simulink model "Transform"  (R2017a)
settings: Solver=VariableStepAuto  StartTime=0.0  StopTime=10.0  MaxStep=0.01  RelTol=1e-3
settings Model: Creator=drone  LastModifiedBy=drone

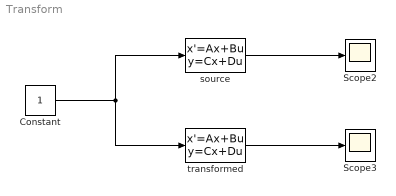
== system Transform ==
  Constant : Constant
  Scope2 : Scope
  Scope3 : Scope
  source : StateSpace  A=[0.5 -10; 1 -2]  B=[0; 1]  C=[3 1]  D=0  X0=0
  transformed : StateSpace  A=[5.5 -1.25; 38 -7]  B=[0; 2]  C=[10 0.5]  D=0  X0=0
  wires:
  Constant/1 -> source/1, transformed/1
  source/1 -> Scope2/1
  transformed/1 -> Scope3/1
